simulink model "aggressive_cascaded_control"  (R2025b)
settings: Solver=VariableStepAuto  StartTime=0.0  StopTime=10.0  RelTol=1e-3
undefined symbols (not defined in the file or in its folder): b_z, G1, G2, J, K_Iw, K_Omega, k_tau, K_xi, Ka, Kv, Kx, m
libraries: eeGeneralControl x3, aerolibutil x2
settings Model: Creator=Gover  LastModifiedBy=Gover

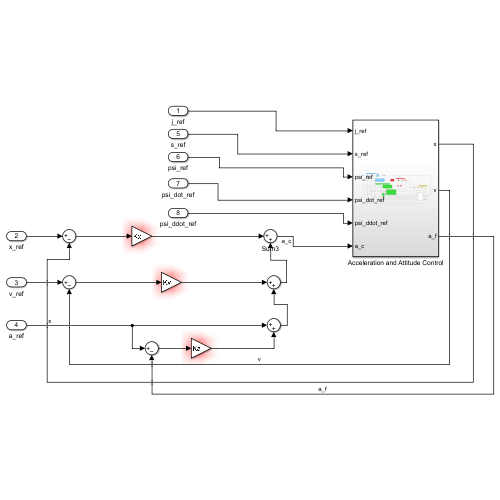
[thumbnail: Simulink's stored preview of the top-level diagram]
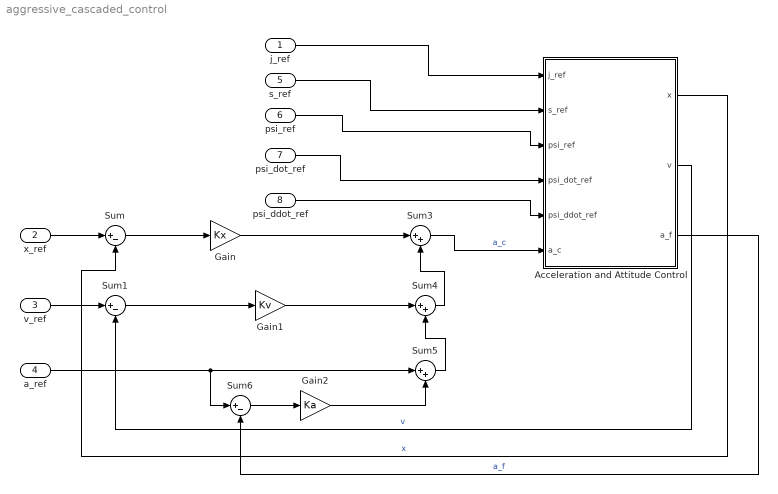
== system aggressive_cascaded_control ==
  j_ref : Inport
  x_ref : Inport  Port=2
  v_ref : Inport  Port=3
  a_ref : Inport  Port=4
  s_ref : Inport  Port=5
  psi_ref : Inport  Port=6
  psi_dot_ref : Inport  Port=7
  psi_ddot_ref : Inport  Port=8
  Acceleration and Attitude Control : Subsystem
  Gain : Gain  Gain=Kx
  Gain1 : Gain  Gain=Kv
  Gain2 : Gain  Gain=Ka
  Sum : Sum  Inputs=|+-
  Sum1 : Sum  Inputs=|+-
  Sum3 : Sum  Inputs=|++
  Sum4 : Sum  Inputs=|++
  Sum5 : Sum  Inputs=|++
  Sum6 : Sum  Inputs=|+-
  wires:
  x_ref/1 -> Sum/1
  Gain/1 -> Sum3/1
  Sum/1 -> Gain/1
  v_ref/1 -> Sum1/1
  Sum1/1 -> Gain1/1
  Gain1/1 -> Sum4/1
  a_ref/1 -> Sum6/1, Sum5/1
  Sum6/1 -> Gain2/1
  Sum3/1 -> Acceleration and Attitude Control/6(a_c)  "a_c"
  Acceleration and Attitude Control/3(a_f) -> Sum6/2  "a_f"
  Gain2/1 -> Sum5/2
  Sum5/1 -> Sum4/2
  Sum4/1 -> Sum3/2
  Acceleration and Attitude Control/2(v) -> Sum1/2  "v"
  Acceleration and Attitude Control/1(x) -> Sum/2  "x"
  j_ref/1 -> Acceleration and Attitude Control/1(j_ref)
  s_ref/1 -> Acceleration and Attitude Control/2(s_ref)
  psi_ref/1 -> Acceleration and Attitude Control/3(psi_ref)
  psi_dot_ref/1 -> Acceleration and Attitude Control/4(psi_dot_ref)
  psi_ddot_ref/1 -> Acceleration and Attitude Control/5(psi_ddot_ref)

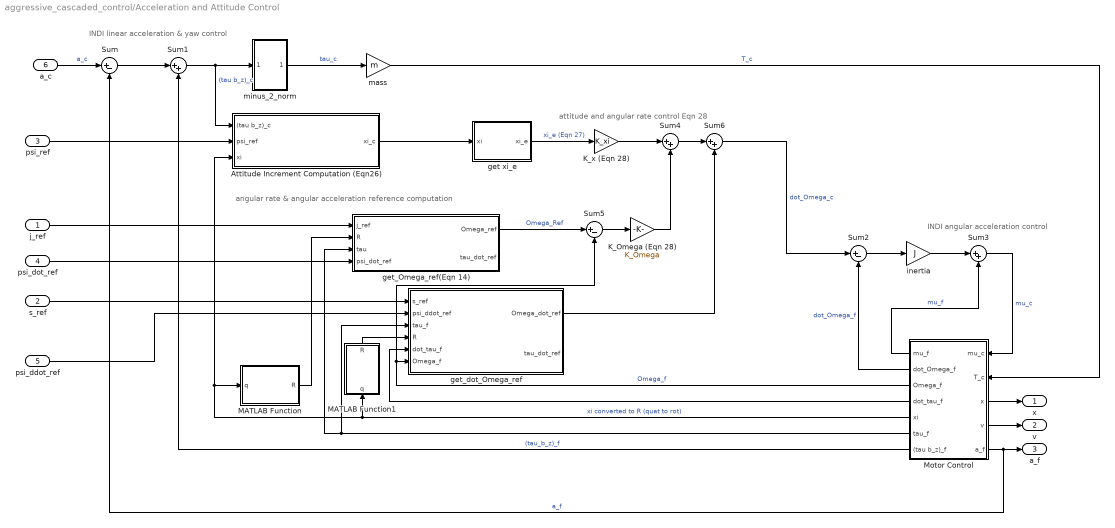
== system aggressive_cascaded_control/Acceleration and Attitude Control ==
  note: attitude and angular rate control Eqn 28
  note: angular rate & angular acceleration reference computation
  note: INDI linear acceleration & yaw control
  note: INDI angular acceleration control
  j_ref : Inport
  s_ref : Inport  Port=2
  psi_ref : Inport  Port=3
  psi_dot_ref : Inport  Port=4
  psi_ddot_ref : Inport  Port=5
  a_c : Inport  Port=6
  Attitude Increment Computation (Eqn26) : Subsystem
  K_Omega (Eqn 28) : Gain  Gain=K_Omega
  K_x (Eqn 28) : Gain  Gain=K_xi
  MATLAB Function : MATLAB Function  TreatAsAtomicUnit=on
  MATLAB Function1 : MATLAB Function  TreatAsAtomicUnit=on
  Motor Control : Subsystem
      settings: PortSchema="{\"entries\":[{\"content\":{\"sides\":[{\"content\":{\"connectorIds\":[\"Out4\",\"Out5\",\"Out6\",\"Out7\",\"Out8\",\"Out9\",\"Out10\"]},\"type\":\"ConnectorPlacement.EquallySpacedRectSide\",\"uuid\":\"f723bf6c-4c67-423b-a9c3-cd0bb2707477\"},{\"content\":{\"connectorIds\":[\"In1\",\"In2\",\"Out1\",\"Out2\",\"Out3\"],\"side\":\"RIGHT\"},\"type\":\"ConnectorPlacement.EquallySpacedRectSide\",\"uuid\":\"19dd196b-8b88-4a00-85ef-e6774b90729c\"},{\"content\":{\"side\":\"TOP\"},\"type\":\"ConnectorPlacement.EquallySpacedRectSide\",\"uuid\":\"0ed846f4-fca4-411c-b5e5-9aee43dcc09b\"}]},\"type\":\"ConnectorPlacement.EquallySpacedConnector\",\"uuid\":\"ef96fbf9-2f29-4429-a371-8bf2634b73a3\"}],\"packageUris\":[\"http://schema.mathworks.com/mf0/Connector/R2020b\"],\"version\":\"1.0\"}"
  Sum : Sum  Inputs=|+-
  Sum{1,3..4,6} (4 alike) : Sum  Inputs=|++
  Sum2 : Sum  Inputs=|+-
  Sum5 : Sum  Inputs=|+-
  get xi_e : MATLAB Function  TreatAsAtomicUnit=on
  get_Omega_ref(Eqn 14) : MATLAB Function  TreatAsAtomicUnit=on
  get_dot_Omega_ref : MATLAB Function  TreatAsAtomicUnit=on
  inertia : Gain  Gain=J
  mass : Gain  Gain=m
  minus_2_norm : Subsystem
  x : Outport
  v : Outport  Port=2
  a_f : Outport  Port=3
  wires:
  a_c/1 -> Sum/1  "a_c"
  Sum/1 -> Sum1/1
  Sum1/1 -> minus_2_norm/1(In1), Attitude Increment Computation (Eqn26)/1((tau b_z)_c)  "(tau b_z)_c"
  minus_2_norm/1(Out1) -> mass/1  "tau_c"
  Motor Control/1(x) -> x/1
  Motor Control/2(v) -> v/1
  Motor Control/3(a_f) -> Sum/2, a_f/1  "a_f"
  Motor Control/5(dot_Omega_f) -> Sum2/2  "dot_Omega_f"
  Sum2/1 -> inertia/1
  inertia/1 -> Sum3/1
  Motor Control/4(mu_f) -> Sum3/2  "mu_f"
  Sum3/1 -> Motor Control/1(mu_c)  "mu_c"
  mass/1 -> Motor Control/2(T_c)  "T_c"
  psi_ref/1 -> Attitude Increment Computation (Eqn26)/2(psi_ref)
  Motor Control/8(xi) -> MATLAB Function1/1(q), MATLAB Function/1(q), Attitude Increment Computation (Eqn26)/3(xi)  "xi converted to R (quat to rot)"
  Motor Control/10((tau b_z)_f) -> Sum1/2  "(tau_b_z)_f"
  MATLAB Function/1(R) -> get_Omega_ref(Eqn 14)/2(R)
  j_ref/1 -> get_Omega_ref(Eqn 14)/1(j_ref)
  psi_dot_ref/1 -> get_Omega_ref(Eqn 14)/4(psi_dot_ref)
  Motor Control/9(tau_f) -> get_Omega_ref(Eqn 14)/3(tau), get_dot_Omega_ref/3(tau_f)
  s_ref/1 -> get_dot_Omega_ref/1(s_ref)
  psi_ddot_ref/1 -> get_dot_Omega_ref/2(psi_ddot_ref)
  Motor Control/7(dot_tau_f) -> get_dot_Omega_ref/5(dot_tau_f)
  Motor Control/6(Omega_f) -> get_dot_Omega_ref/6(Omega_f), Sum5/2  "Omega_f"
  MATLAB Function1/1(R) -> get_dot_Omega_ref/4(R)
  Attitude Increment Computation (Eqn26)/1(xi_c) -> get xi_e/1(xi)
  get xi_e/1(xi_e) -> K_x (Eqn 28)/1  "xi_e (Eqn 27)"
  K_x (Eqn 28)/1 -> Sum4/1
  get_Omega_ref(Eqn 14)/1(Omega_ref) -> Sum5/1  "Omega_Ref"
  Sum5/1 -> K_Omega (Eqn 28)/1
  K_Omega (Eqn 28)/1 -> Sum4/2
  Sum4/1 -> Sum6/1
  get_dot_Omega_ref/1(Omega_dot_ref) -> Sum6/2
  Sum6/1 -> Sum2/1  "dot_Omega_c"

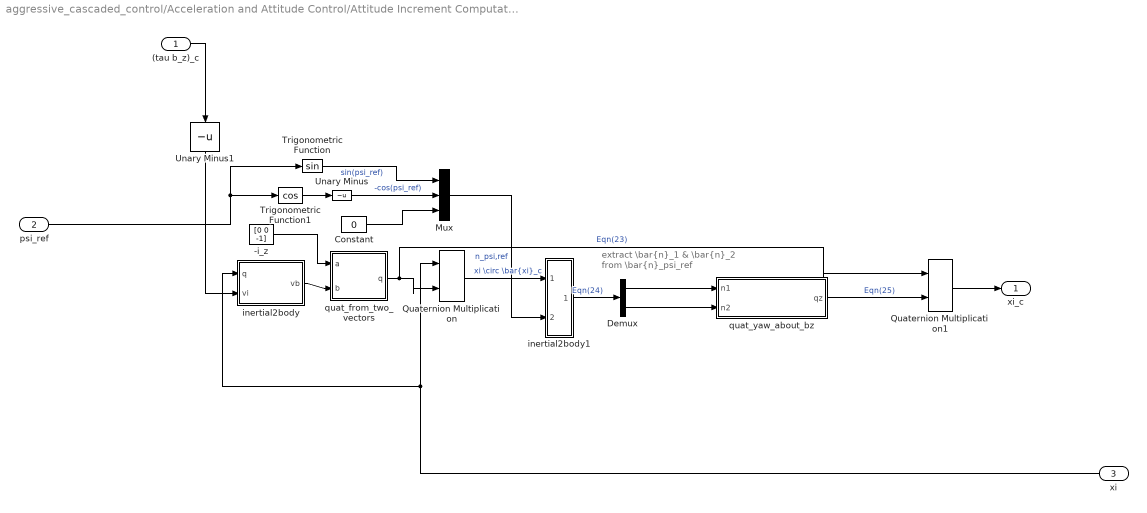
== system aggressive_cascaded_control/Acceleration and Attitude Control/Attitude Increment Computation (Eqn26) ==
  note: extract \bar{n}_1 & \bar{n}_2 from \bar{n}_psi_ref
  (tau b_z)_c : Inport
  psi_ref : Inport  Port=2
  xi : Inport  Port=3
  " quat_from_two_vectors" : MATLAB Function  TreatAsAtomicUnit=on
  -i_z : Constant  Value=[0 0 -1]
  Constant : Constant  Value=0
  Demux : Demux  Outputs=2
  Mux : Mux  Inputs=3
  Quaternion Multiplication : aerolibutil/Quaternion Multiplication
  Quaternion Multiplication1 : aerolibutil/Quaternion Multiplication
  Trigonometric Function : Trigonometry
  Trigonometric Function1 : Trigonometry  Operator=cos
  Unary Minus : UnaryMinus
  Unary Minus1 : UnaryMinus
  inertial2body : MATLAB Function  TreatAsAtomicUnit=on
  inertial2body1 : MATLAB Function  TreatAsAtomicUnit=on
  quat_yaw_about_bz : MATLAB Function  TreatAsAtomicUnit=on
  xi_c : Outport
  wires:
  inertial2body/1(vb) -> " quat_from_two_vectors"/2(b)
  Demux/2 -> quat_yaw_about_bz/2(n2)
  (tau b_z)_c/1 -> Unary Minus1/1
  Constant/1 -> Mux/3
  psi_ref/1 -> Trigonometric Function/1, Trigonometric Function1/1
  " quat_from_two_vectors"/1(q) -> Quaternion Multiplication/2, Quaternion Multiplication1/1  "Eqn(23)"
  Trigonometric Function1/1 -> Unary Minus/1
  Unary Minus/1 -> Mux/2  "-cos(psi_ref)"
  Trigonometric Function/1 -> Mux/1  "sin(psi_ref)"
  Unary Minus1/1 -> inertial2body/2(vi)
  Quaternion Multiplication/1 -> inertial2body1/1(q)  "xi \\circ \\bar{xi}_c"
  quat_yaw_about_bz/1(qz) -> Quaternion Multiplication1/2  "Eqn(25)"
  xi/1 -> inertial2body/1(q), Quaternion Multiplication/1
  -i_z/1 -> " quat_from_two_vectors"/1(a)
  Mux/1 -> inertial2body1/2(vi)  "n_psi,ref"
  inertial2body1/1(vb) -> Demux/1  "Eqn(24)"
  Quaternion Multiplication1/1 -> xi_c/1
  Demux/1 -> quat_yaw_about_bz/1(n1)

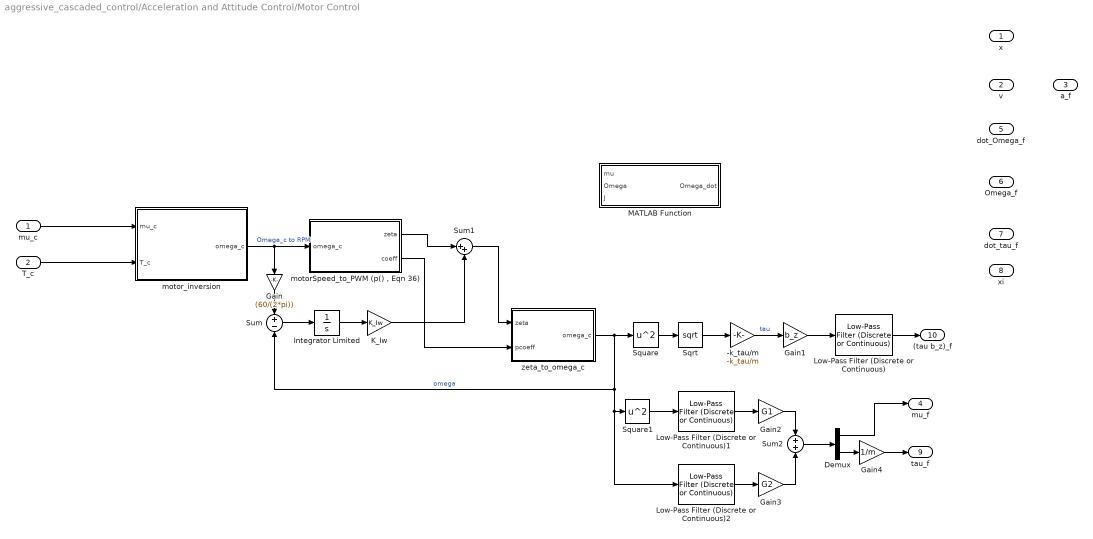
== system aggressive_cascaded_control/Acceleration and Attitude Control/Motor Control ==
  mu_c : Inport
  T_c : Inport  Port=2
  -k_tau/m : Gain  Gain=-k_tau/m
  Demux : Demux  Outputs=2
  Gain : Gain  Gain=(60/(2*pi))
  Gain1 : Gain  Gain=b_z
  Gain2 : Gain  Gain=G1
  Gain3 : Gain  Gain=G2
  Gain4 : Gain  Gain=1/m
  Integrator Limited : Integrator  LimitOutput=on  UpperSaturationLimit=22598  LowerSaturationLimit=0
  K_Iw : Gain  Gain=K_Iw
  Low-Pass Filter (Discrete or Continuous) : eeGeneralControl/Low-Pass Filter (Discrete or Continuous)  K=1  T=1  B=inf  A=-inf  init_option=Inherited from block input  x0=0  Ts=-1
  Low-Pass Filter (Discrete or Continuous)1 : eeGeneralControl/Low-Pass Filter (Discrete or Continuous)  K=1  T=1  B=inf  A=-inf  init_option=Inherited from block input  x0=0  Ts=-1
  Low-Pass Filter (Discrete or Continuous)2 : eeGeneralControl/Low-Pass Filter (Discrete or Continuous)  K=1  T=1  B=inf  A=-inf  init_option=Inherited from block input  x0=0  Ts=-1
  MATLAB Function : MATLAB Function  TreatAsAtomicUnit=on
  Sqrt : Sqrt
  Square : Math  Operator=square
  Square1 : Math  Operator=square
  Sum : Sum  Inputs=+|-
  Sum1 : Sum  Inputs=|++
  Sum2 : Sum  Inputs=+|+
  "motorSpeed_to_PWM (p() , Eqn 36)" : MATLAB Function  TreatAsAtomicUnit=on
  motor_inversion : MATLAB Function  TreatAsAtomicUnit=on
  zeta_to_omega_c : MATLAB Function  TreatAsAtomicUnit=on
  x : Outport
  v : Outport  Port=2
  a_f : Outport  Port=3
  mu_f : Outport  Port=4
  dot_Omega_f : Outport  Port=5
  Omega_f : Outport  Port=6
  dot_tau_f : Outport  Port=7
  xi : Outport  Port=8
  tau_f : Outport  Port=9
  (tau b_z)_f : Outport  Port=10
  wires:
  mu_c/1 -> motor_inversion/1(mu_c)
  T_c/1 -> motor_inversion/2(T_c)
  motor_inversion/1(omega_c) -> "motorSpeed_to_PWM (p() , Eqn 36)"/1(omega_c), Gain/1  "Omega_c to RPM"
  Sum/1 -> Integrator Limited/1
  Integrator Limited/1 -> K_Iw/1
  "motorSpeed_to_PWM (p() , Eqn 36)"/1(zeta) -> Sum1/1
  K_Iw/1 -> Sum1/2
  Gain/1 -> Sum/1
  "motorSpeed_to_PWM (p() , Eqn 36)"/2(coeff) -> zeta_to_omega_c/2(pcoeff)
  Sum1/1 -> zeta_to_omega_c/1(zeta)
  zeta_to_omega_c/1(omega_c) -> Sum/2, Low-Pass Filter (Discrete or Continuous)2/1, Square1/1, Square/1  "omega"
  Square/1 -> Sqrt/1
  Sqrt/1 -> -k_tau/m/1
  -k_tau/m/1 -> Gain1/1  "tau"
  Gain1/1 -> Low-Pass Filter (Discrete or Continuous)/1
  Low-Pass Filter (Discrete or Continuous)/1 -> (tau b_z)_f/1
  Square1/1 -> Low-Pass Filter (Discrete or Continuous)1/1
  Low-Pass Filter (Discrete or Continuous)1/1 -> Gain2/1
  Low-Pass Filter (Discrete or Continuous)2/1 -> Gain3/1
  Gain2/1 -> Sum2/1
  Gain3/1 -> Sum2/2
  Sum2/1 -> Demux/1
  Demux/1 -> mu_f/1
  Demux/2 -> Gain4/1
  Gain4/1 -> tau_f/1

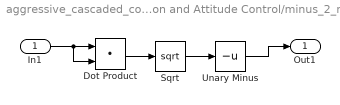
== system aggressive_cascaded_control/Acceleration and Attitude Control/minus_2_norm ==
  In1 : Inport
  Dot Product : DotProduct  OutDataTypeStr=Inherit: Inherit via internal rule
  Sqrt : Sqrt
  Unary Minus : UnaryMinus
  Out1 : Outport
  wires:
  Unary Minus/1 -> Out1/1
  In1/1 -> Dot Product/2, Dot Product/1
  Dot Product/1 -> Sqrt/1
  Sqrt/1 -> Unary Minus/1

== matlab function aggressive_cascaded_control/Acceleration and Attitude Control/Motor Control/zeta_to_omega_c ==
  data: zeta input; omega_c output; pcoeff input
function omega_c = p_inv(zeta, pcoeff)
% pcoeff: polynomial coeffs for zeta = p(omega)
omega_c = zeros(4,1);
for i=1:4
    c = pcoeff(i,:);           % [a2 a1 a0] or [a3 a2 a1 a0]
    % initial guess (scale ζ by table limits)
    w0 = 20000*zeta(i);
    f  = @(w) polyval(c,w) - zeta(i);
    omega_c(i) = fzero(f, max(1,w0));
end
end

== matlab function aggressive_cascaded_control/Acceleration and Attitude Control/Motor Control/MATLAB Function ==
  data: mu input; Omega_dot output; Omega input; J input
function Omega_dot = omega_dot(mu, Omega, J)
Omega_dot = J \ (mu - cross(Omega, J*Omega));
end

== matlab function aggressive_cascaded_control/Acceleration and Attitude Control/Attitude Increment Computation (Eqn26)/ quat_from_two_vectors ==
  data: a input; q output; b input
function q = quat_from_two_vectors(a,b)
% a,b 3x1 or 1x3, assumed unit
a = a(:)/norm(a); b = b(:)/norm(b);
w = 1 + dot(a,b);
v = cross(a,b);
if w < 1e-6         % nearly 180 deg: pick any axis ⟂ a
    w = 0;
    % for a = [0;0;-1], an easy orthogonal axis:
    v = [1;0;0];
end
q = [w; v];         % [w;x;y;z]
q = q / norm(q);
q = q.';            % row for Simulink consistency
end

== matlab function aggressive_cascaded_control/Acceleration and Attitude Control/Attitude Increment Computation (Eqn26)/inertial2body ==
  data: q input; vb output; vi input
function vb = inertial2body(q, vi)
% vb = inertial2body(q, vi)
% Rotates inertial-frame vector vi into the body frame using quaternion q
% q: 1x4 or 4x1 quaternion [w x y z] (body→inertial)
% vi: 1x3 or 3x1 vector in inertial frame
% Output vb: 1x3 normalized vector in body frame

% Ensure row vector orientation
if size(q,1) > 1, q = q.'; end
if size(vi,1) > 1, vi = vi.'; end

% Rotate inertial → body
qc = quatconj(q);          % conjugate = inverse rotation
vb = quatrotate(qc, vi);   % rotate vi into body frame

% Normalize to unit length (avoid divide-by-zero)
n = norm(vb);
if n > 1e-9
    vb = vb / n;
else
    vb = [0 0 0];  % fallback if degenerate
end
end

== matlab function aggressive_cascaded_control/Acceleration and Attitude Control/Attitude Increment Computation (Eqn26)/inertial2body1 ==
  data: q input; vb output; vi input
function vb = inertial2body(q, vi)
% vb = inertial2body(q, vi)
% Rotates inertial-frame vector vi into the body frame using quaternion q
% q: 1x4 or 4x1 quaternion [w x y z] (body→inertial)
% vi: 1x3 or 3x1 vector in inertial frame
% Output vb: 1x3 normalized vector in body frame
vi = -vi; %we need (-bz)^b_c
% Ensure row vector orientation
if size(q,1) > 1, q = q.'; end
if size(vi,1) > 1, vi = vi.'; end

% Rotate inertial → body
qc = quatconj(q);          % conjugate = inverse rotation
vb = quatrotate(qc, vi);   % rotate vi into body frame

% Normalize to unit length (avoid divide-by-zero)
n = norm(vb);
if n > 1e-9
    vb = vb / n;
else
    vb = [0 0 0];  % fallback if degenerate
end
end

== matlab function aggressive_cascaded_control/Acceleration and Attitude Control/Attitude Increment Computation (Eqn26)/quat_yaw_about_bz ==
  data: n1 input; n2 input; qz output
function qz = quat_yaw_about_bz(n1,n2)
q = [1 0 0 -n1/n2];
qz = qz / norm(qz);
end

== matlab function aggressive_cascaded_control/Acceleration and Attitude Control/get_Omega_ref(Eqn 14) ==
  data: j_ref input; R input; tau input; Omega_ref output; psi_dot_ref input; tau_dot_ref output
function [Omega_ref, tau_dot_ref] = get_Omega_ref(j_ref, R, tau, psi_dot_ref)

% Columns of R are body axes in inertial frame
bx = R(:,1);  by = R(:,2);  bz = R(:,3);

% r_psi = [b_x^1; b_x^2; 0]
rpsi = [bx(1); bx(2); 0];
den  = rpsi(1)^2 + rpsi(2)^2;       % r_psi^T r_psi
% Guard for near-degenerate case
if den < 1e-9
    % fallback (e.g., keep previous S or set S=[0 0 0])
    S = [0 0 0];
else
    s1 = [-bx(2), bx(1)] / den;     % 1x2
    s2 = [ 0, -bz(1),  by(1);       % 2x3
           0, -bz(2),  by(2) ];
    S  = s1 * s2;                   % 1x3
end

% Skew of i_z = [0;0;1]
Skew = [ 0 -1  0;
         1  0  0;
         0  0  0 ];
% Note: [i_z]_x is skew-symmetric ⇒ ([i_z]_x)^T = -[i_z]_x
A11 = tau * (R * Skew');             % = -tau * R * Skew (3x3)
A12 = bz;                            % 3x1
A21 = S;                             % 1x3
A22 = 0;                             % 1x1

A = [A11, A12; A21, A22];            % 4x4
b = [j_ref(:); psi_dot_ref];         % 4x1

x = A \ b;                           % solve
Omega_ref   = x(1:3);
tau_dot_ref = x(4);
end

== matlab function aggressive_cascaded_control/Acceleration and Attitude Control/MATLAB Function ==
  data: q input; R output
function R = quad_to_rot(q)
w = q(1);
x = q(2);
y = q(3);
z = q(4);
% If you have Robotics System Toolbox:
R = quat2rotm([w x y z]);     % scalar-first

% Or using the quaternion class (R2020a+):
q = quaternion(w,x,y,z);      % scalar-first ctor
R = rotmat(q,'frame');        % body->inertial; use 'point' for inertial->body

% Older Aerospace Toolbox:
R = quat2dcm([w x y z]);      % deprecated name, same convention

end

== matlab function aggressive_cascaded_control/Acceleration and Attitude Control/get_dot_Omega_ref ==
  data: s_ref input; psi_ddot_ref input; tau_f input; Omega_dot_ref output; R input; tau_dot_ref output; dot_tau_f input; Omega_f input
function [Omega_dot_ref, tau_dot_ref] = get_dot_Omega_ref( ...
    s_ref, psi_ddot_ref, tau_f, R, dot_tau_f, Omega_f)

% Columns of R are body axes in inertial frame
bx = R(:,1);  by = R(:,2);  bz = R(:,3);

% r_psi = [b_x^1; b_x^2; 0]
rpsi = [bx(1); bx(2); 0];
den  = rpsi(1)^2 + rpsi(2)^2;       % r_psi^T r_psi

% Build S and Sdot
if den < 1e-9
    S = [0 0 0];     % robust fallback near singular projection
    Sdot = [0 0 0];
else
    % S = s1 * s2 where
    s1 = [-bx(2), bx(1)] / den;                   % 1x2
    s2 = [ 0, -bz(1),  by(1);                     % 2x3
           0, -bz(2),  by(2) ];
    S  = s1 * s2;                                 % 1x3

    % time-derivatives via bdot = Ω × b  (Ω in body, b in inertial)
    bx_dot = cross(Omega_f, bx);
    by_dot = cross(Omega_f, by);
    bz_dot = cross(Omega_f, bz);

    % den_dot = 2 rpsi^T rpsi_dot
    rpsi_dot = [bx_dot(1); bx_dot(2); 0];
    den_dot  = 2 * (rpsi(1)*rpsi_dot(1) + rpsi(2)*rpsi_dot(2));   % scalar

    % s1_dot by product rule
    s1_dot = ([-bx_dot(2), bx_dot(1)] / den) - (s1 * (den_dot/den));

    % s2_dot from by_dot, bz_dot
    s2_dot = [ 0, -bz_dot(1),  by_dot(1);
               0, -bz_dot(2),  by_dot(2) ];

    % Sdot
    Sdot = s1_dot * s2 + s1 * s2_dot;            % 1x3
end

% Skew of i_z = [0;0;1]
Skew_iz = [ 0 -1  0;
            1  0  0;
            0  0  0 ];

% [Ω]_x
skew_Omega = [   0       -Omega_f(3)  Omega_f(2);
               Omega_f(3)   0         -Omega_f(1);
              -Omega_f(2)  Omega_f(1)   0       ];

% Left-hand matrix in (15): [ τ R [i_z]_x^T   bz ;  S   0 ]
A11 = tau_f * (R * Skew_iz');                   % = -tau_f * R * Skew_iz
A12 = bz;
A21 = S;
A22 = 0;
A = [A11, A12; A21, A22];                       % 4x4

% Right-hand vector in (15): [s_ref ; psi_ddot_ref] - [ R(2 dotτ I + τ [Ω]_x)[i_z]_x^T Ω ; Sdot Ω ]
btop = s_ref - R * ( 2*dot_tau_f*eye(3) + tau_f*skew_Omega ) * (Skew_iz') * Omega_f;
bbot = psi_ddot_ref - Sdot * Omega_f;
b    = [btop; bbot];

% Solve
x = A \ b;
Omega_dot_ref = x(1:3);
tau_dot_ref   = x(4);
end

== matlab function aggressive_cascaded_control/Acceleration and Attitude Control/MATLAB Function1 ==
  data: q input; R output
function R = quad_to_rot(q)
w = q(1);
x = q(2);
y = q(3);
z = q(4);
% If you have Robotics System Toolbox:
R = quat2rotm([w x y z]);     % scalar-first

% Or using the quaternion class (R2020a+):
q = quaternion(w,x,y,z);      % scalar-first ctor
R = rotmat(q,'frame');        % body->inertial; use 'point' for inertial->body

% Older Aerospace Toolbox:
R = quat2dcm([w x y z]);      % deprecated name, same convention

end

== matlab function aggressive_cascaded_control/Acceleration and Attitude Control/get xi_e ==
  data: xi input; xi_e output
function xi_e = error_angle(xi)
w = xi(1);
x = xi(2);
y = xi(3);
z = xi(4);
xi_e = 2*arccos(q)/(sqrt(1-w*w)) * [x y z]';
% eqn (27)



end

== matlab function aggressive_cascaded_control/Acceleration and Attitude Control/Motor Control/motor_inversion ==
  data: mu_c input; omega_c output; T_c input
function omega_c = fcn(mu_c, T_c)


ly = 0.3;
lx = 0.3;
k_tau = 0.01;
k_mu_z = 0.01;
G1 = [ly*k_tau -ly*k_tau -ly*k_tau ly*k_tau;
     lx*k_tau lx*k_tau -lx*k_tau -lx*k_tau;
     -k_mu_z k_mu_z -k_mu_z k_mu_z;
     -k_tau -k_tau -k_tau -k_tau];


omega_c = sqrt(inv(G1)*[mu_c;T_c]);

end

== matlab function aggressive_cascaded_control/Acceleration and Attitude Control/Motor Control/motorSpeed_to_PWM (p() , Eqn 36) ==
  data: omega_c input; zeta output; coeff output
function [zeta, coeff]= p_of_omega(omega_c)
    % p_of_omega  Map commanded motor speeds → throttle commands (normalized)
    %
    %   zeta = p_of_omega(omega_c)  
    %
    %   Inputs:
    %     omega_c  – Nx1 (or 4x1) vector of commanded motor speeds (in RPM)
    %
    %   Outputs:
    %     zeta     – Nx1 (or 4x1) vector of normalized throttle commands [0,1]
    %
    %   Notes:
    %     - Based on empirical table from Bitcraze “PWM to Thrust / RPM” data. :contentReference[oaicite:1]{index=1}
    %     - Uses a degree-2 polynomial fit: ζ = a0 + a1*ω + a2*ω^2
    %     - ω units: RPM. If you use rad/s, convert accordingly: RPM = (60/(2π)) * ω_rad_s
    %     - Output is saturated to [0,1].
    %
    %   Example:
    %     omega_vec = [10000; 15000; 20000; 22000];
    %     zeta_vec  = p_of_omega(omega_vec);
    
    % Calibration data (RPM vs normalized throttle ζ = PWM%/100)
    % From Bitcraze page: PWM % vs RPM (stock Crazyflie 2.x) :contentReference[oaicite:2]{index=2}
    omega_c =  (60/(2*pi)) * omega_c;
    RPM_data = [ ...
         0;
         4485;
         7570;
         9374;
        10885;
        12277;
        13522;
        14691;
        15924;
        17174;
        18179;
        19397;
        20539;
        21692;
        22598;
        23882
        ];
    PWM_pct_data = [ ...
         0.00;
         6.25;
        12.50;
        18.75;
        25.00;
        31.25;
        37.50;
        43.25;
        50.00;
        56.25;
        62.50;
        68.75;
        75.00;
        81.25;
        87.50;
    	93.75
        ];
    zeta_data = PWM_pct_data / 100;  % normalize to [0,1]
    
    % Fit degree-2 polynomial: ζ ≈ a0 + a1*ω + a2*ω^2
    degree = 2;
    p = polyfit(RPM_data, zeta_data, degree);
    % p(1)*ω^2 + p(2)*ω + p(3)
    coeff = p;
    % Evaluate for input omega_c
    zeta = polyval(p, omega_c);
    
    % Saturate between 0 and 1
    zeta(zeta < 0) = 0;
    zeta(zeta > 1) = 1;
end
